simulink model "UDP_Model"  (R2016b)
settings: Solver=FixedStepDiscrete  StartTime=0.0  StopTime=inf  RelTol=1e-3  EnableMultiTasking=on
InitFcn:
  | RIEKF_InitFcn;
libraries: UDP_Communication x4
settings Model: xpc_rtwmakecfg_data=_xpcethercatlib_  ParamWorkspaceSource=ReferencedWorkspace  Creator=robot  LastModifiedBy=Ross Hartley
settings SolverCC: EnableConcurrentExecution=on  ConcurrentTasks=on
settings DataIOCC: SaveFormat=Array  SaveOutput=off  SignalLogging=off  DSMLogging=off  VisualizeSimOutput=off  SaveTime=off
settings OptimizationCC: DefaultParameterBehavior=Inlined  InlineInvariantSignals=on  LifeSpan=inf  SimCompilerOptimization=on  AccelVerboseBuild=on
settings DebuggingCC: AllowSymbolicDim=off  SFUnexpectedBacktrackingDiag=warning  SFNoUnconditionalDefaultTransitionDiag=warning  SFExecutionAtInitializationDiag=none
settings HardwareCC: ProdBitPerPointer=32  ProdBitPerSizeT=32  ProdBitPerPtrDiffT=32  ProdLargestAtomicFloat=None  ProdWordSize=32  ProdLongLongMode=on  ProdHWDeviceType=Generic->32-bit x86 compatible
settings ModelReferenceCC: ParallelModelReferenceMATLABWorkerInit=Copy Base Workspace  ModelReferenceNumInstancesAllowed=Single
settings SFSimCC: SFSimEcho=off
settings RTWCC: SystemTargetFile=slrt.tlc  TLCOptions=-axPCMaxOverloads=1000000000 -axPCMaxOverloadLen=1000000000  TemplateMakefile=slrt_default_tmf  Description=Simulink Real-Time  RTWUseSimCustomCode=on  CodeExecutionProfiling=on  RTWCompilerOptimization=on
settings CodeAppCC: GenerateComments=off  MaxIdLength=128  SimulinkBlockComments=off
settings SimulinkRealTimeCC: ExtMode=off
settings ConfigComp: CovMetricSettings=dw  CovHtmlReporting=on  CovSaveCumulativeToWorkspaceVar=on  CovSaveSingleToWorkspaceVar=on  CovExternalEMLEnable=off

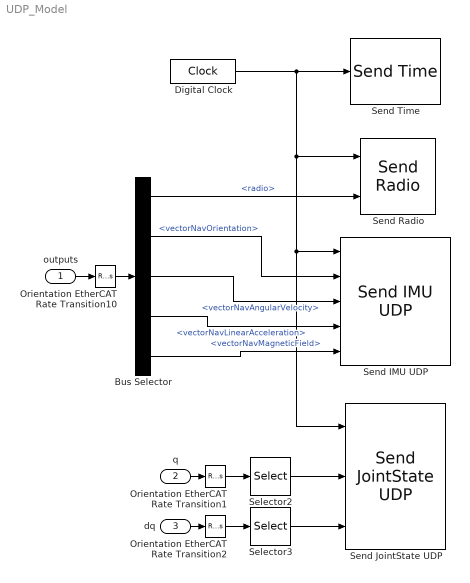
== system UDP_Model ==
  outputs : Inport  OutDataTypeStr=Bus: cassieOutputsBus  BusOutputAsStruct=on
  q : Inport  Port=2
  dq : Inport  Port=3
  Bus Selector : BusSelector  OutputSignals=radio,vectorNavOrientation,vectorNavAngularVelocity,vectorNavLinearAcceleration,vectorNavMagneticField
  Digital Clock : DigitalClock  SampleTime=-1
  Orientation EtherCAT Rate Transition1 : RateTransition  Deterministic=off  OutPortSampleTime=UDP_SampleTime
  Orientation EtherCAT Rate Transition10 : RateTransition  Deterministic=off  OutPortSampleTime=UDP_SampleTime
  Orientation EtherCAT Rate Transition2 : RateTransition  Deterministic=off  OutPortSampleTime=UDP_SampleTime
  Selector2 : Selector  InputPortWidth=20  IndexOptions=Index vector (dialog)  Indices=[7:20]  OutputSizes=1
  Selector3 : Selector  InputPortWidth=20  IndexOptions=Index vector (dialog)  Indices=[7:20]  OutputSizes=1
  Send IMU UDP : UDP_Communication/Send IMU UDP
  Send JointState UDP : UDP_Communication/Send JointState UDP
  Send Radio : UDP_Communication/Send Radio
  Send Time : UDP_Communication/Send Time
  wires:
  Digital Clock/1 -> Send JointState UDP/1, Send IMU UDP/1, Send Radio/1, Send Time/1
  Selector3/1 -> Send JointState UDP/3
  Selector2/1 -> Send JointState UDP/2
  outputs/1 -> Orientation EtherCAT Rate Transition10/1
  Bus Selector/1 -> Send Radio/2  "<radio>"
  Bus Selector/2 -> Send IMU UDP/2  "<vectorNavOrientation>"
  Bus Selector/3 -> Send IMU UDP/3  "<vectorNavAngularVelocity>"
  Bus Selector/4 -> Send IMU UDP/4  "<vectorNavLinearAcceleration>"
  Bus Selector/5 -> Send IMU UDP/5  "<vectorNavMagneticField>"
  Orientation EtherCAT Rate Transition10/1 -> Bus Selector/1
  dq/1 -> Orientation EtherCAT Rate Transition2/1
  Orientation EtherCAT Rate Transition2/1 -> Selector3/1
  q/1 -> Orientation EtherCAT Rate Transition1/1
  Orientation EtherCAT Rate Transition1/1 -> Selector2/1
